simulink model "FSAC2021"  (R2014a)
settings: Solver=FixedStepDiscrete  StartTime=0.0  StopTime=inf  FixedStep=0.0005  RelTol=1e-3
model workspace (MAT data in the model file):
  MCOS : class17 (value not decoded)
  MCOS : class17 (value not decoded)
  MCOS : class17 (value not decoded)
  MCOS : class17 (value not decoded)
  MCOS : class17 (value not decoded)
  MCOS : class17 (value not decoded)
  MCOS : class17 (value not decoded)
  MCOS : class17 (value not decoded)
  MCOS : class17 (value not decoded)
  MCOS : class17 (value not decoded)
  MCOS : class17 (value not decoded)
  MCOS : class17 (value not decoded)
  MCOS : class17 (value not decoded)
  MCOS : class17 (value not decoded)
  MCOS : class17 (value not decoded)
  MCOS : class17 (value not decoded)
  MCOS : class17 (value not decoded)
  MCOS : class17 (value not decoded)
  MCOS : class17 (value not decoded)
  BUZZER_START = 1
  MCOS : class17 (value not decoded)
  MCOS : class17 (value not decoded)
  MCOS : class17 (value not decoded)
  MCOS : class17 (value not decoded)
  MCOS : class17 (value not decoded)
  MCOS : class17 (value not decoded)
  MCOS : class17 (value not decoded)
  MCOS : class17 (value not decoded)
  MCOS : class17 (value not decoded)
  MCOS : class17 (value not decoded)
  MCOS : class17 (value not decoded)
  MCOS : class17 (value not decoded)
  MCOS : class17 (value not decoded)
  MCOS : class17 (value not decoded)
  MCOS : class17 (value not decoded)
  MCOS : class17 (value not decoded)
  MCOS : class17 (value not decoded)
  MCOS : class17 (value not decoded)
  MCOS : class17 (value not decoded)
  MCOS : class17 (value not decoded)
  MCOS : class17 (value not decoded)
  MCOS : class17 (value not decoded)
  MCOS : class17 (value not decoded)
  MCOS : class17 (value not decoded)
  MCOS : class17 (value not decoded)
  MCOS : class17 (value not decoded)
  MCOS : class17 (value not decoded)
  MCOS : class17 (value not decoded)
  MCOS : class17 (value not decoded)
  MCOS : class17 (value not decoded)
  MCOS : class17 (value not decoded)
  MCOS : class17 (value not decoded)
  MCOS : class17 (value not decoded)
  MCOS : class17 (value not decoded)
  MCOS : class17 (value not decoded)
  MCOS : class17 (value not decoded)
  MCOS : class17 (value not decoded)
  MCOS : class17 (value not decoded)
  Brake = 11
  MCOS : class17 (value not decoded)
  MCOS : class17 (value not decoded)
  MCOS : class17 (value not decoded)
  MCOS : class17 (value not decoded)
  MCOS : class17 (value not decoded)
  MCOS : class17 (value not decoded)
  MCOS : class17 (value not decoded)
  MCOS : class17 (value not decoded)
  Sensor_Acc_b = 101.85
  Sensor_Acc_k = -0.0185
  Str_Sen_Orig_Angle = -341
  MCOS : class17 (value not decoded)
  Tire_D = 0.47
  T = 0.05
libraries: simulink x396, ec55xxlib x126
(part 8 of 17)

== system FSAC2021/CAN_SEND/Subsystem1/MOTEC_ENCODER1/Str_Encoder1 ==
  Str_Encoder1 : Inport
  Str_Encoder1Ron : Rounding  Operator=round
  Str_Encoder1_1sat : Saturate  UpperLimit=255  LowerLimit=0
  Str_Encoder1_Convert : DataTypeConversion  OutDataTypeStr=uint8
  Str_Encoder1_Convert1 : DataTypeConversion  OutDataTypeStr=uint32
  Str_Encoder1_D : Product  Inputs=*/
  Str_Encoder1_F : Constant  OutDataTypeStr=single
  Str_Encoder1_L : simulink/Logic and Bit Operations/Bitwise Operator  logicop=AND  UseBitMask=on  BitMask=255  BitMaskRealWorld=Stored Integer
  Str_Encoder1_O : Constant  Value=0  OutDataTypeStr=single
  Str_Encoder1_S : ArithShift
  Str_Encoder1_sat : Saturate  UpperLimit=255  LowerLimit=0
  Str_Encoder1_st : Sum  Inputs=+-
  output1 : Outport
  wires:
  Str_Encoder1/1 -> Str_Encoder1_sat/1
  Str_Encoder1_sat/1 -> Str_Encoder1_st/1
  Str_Encoder1_O/1 -> Str_Encoder1_st/2
  Str_Encoder1_st/1 -> Str_Encoder1_D/1
  Str_Encoder1_F/1 -> Str_Encoder1_D/2
  Str_Encoder1_D/1 -> Str_Encoder1Ron/1
  Str_Encoder1Ron/1 -> Str_Encoder1_S/1
  Str_Encoder1_S/1 -> Str_Encoder1_1sat/1
  Str_Encoder1_1sat/1 -> Str_Encoder1_Convert1/1
  Str_Encoder1_Convert1/1 -> Str_Encoder1_L/1
  Str_Encoder1_L/1 -> Str_Encoder1_Convert/1
  Str_Encoder1_Convert/1 -> output1/1

== system FSAC2021/CAN_SEND/Subsystem1/MOTEC_ENCODER1/Str_Encoder2 ==
  Str_Encoder2 : Inport
  Str_Encoder2Ron : Rounding  Operator=round
  Str_Encoder2_1sat : Saturate  UpperLimit=255  LowerLimit=0
  Str_Encoder2_Convert : DataTypeConversion  OutDataTypeStr=uint8
  Str_Encoder2_Convert1 : DataTypeConversion  OutDataTypeStr=uint32
  Str_Encoder2_D : Product  Inputs=*/
  Str_Encoder2_F : Constant  OutDataTypeStr=single
  Str_Encoder2_L : simulink/Logic and Bit Operations/Bitwise Operator  logicop=AND  UseBitMask=on  BitMask=255  BitMaskRealWorld=Stored Integer
  Str_Encoder2_O : Constant  Value=0  OutDataTypeStr=single
  Str_Encoder2_S : ArithShift
  Str_Encoder2_sat : Saturate  UpperLimit=255  LowerLimit=0
  Str_Encoder2_st : Sum  Inputs=+-
  output2 : Outport
  wires:
  Str_Encoder2/1 -> Str_Encoder2_sat/1
  Str_Encoder2_sat/1 -> Str_Encoder2_st/1
  Str_Encoder2_O/1 -> Str_Encoder2_st/2
  Str_Encoder2_st/1 -> Str_Encoder2_D/1
  Str_Encoder2_F/1 -> Str_Encoder2_D/2
  Str_Encoder2_D/1 -> Str_Encoder2Ron/1
  Str_Encoder2Ron/1 -> Str_Encoder2_S/1
  Str_Encoder2_S/1 -> Str_Encoder2_1sat/1
  Str_Encoder2_1sat/1 -> Str_Encoder2_Convert1/1
  Str_Encoder2_Convert1/1 -> Str_Encoder2_L/1
  Str_Encoder2_L/1 -> Str_Encoder2_Convert/1
  Str_Encoder2_Convert/1 -> output2/1

== system FSAC2021/CAN_SEND/Subsystem1/MOTEC_ENCODER1/Str_Encoder3 ==
  Str_Encoder3 : Inport
  Str_Encoder3Ron : Rounding  Operator=round
  Str_Encoder3_1sat : Saturate  UpperLimit=255  LowerLimit=0
  Str_Encoder3_Convert : DataTypeConversion  OutDataTypeStr=uint8
  Str_Encoder3_Convert1 : DataTypeConversion  OutDataTypeStr=uint32
  Str_Encoder3_D : Product  Inputs=*/
  Str_Encoder3_F : Constant  OutDataTypeStr=single
  Str_Encoder3_L : simulink/Logic and Bit Operations/Bitwise Operator  logicop=AND  UseBitMask=on  BitMask=255  BitMaskRealWorld=Stored Integer
  Str_Encoder3_O : Constant  Value=0  OutDataTypeStr=single
  Str_Encoder3_S : ArithShift
  Str_Encoder3_sat : Saturate  UpperLimit=255  LowerLimit=0
  Str_Encoder3_st : Sum  Inputs=+-
  output3 : Outport
  wires:
  Str_Encoder3/1 -> Str_Encoder3_sat/1
  Str_Encoder3_sat/1 -> Str_Encoder3_st/1
  Str_Encoder3_O/1 -> Str_Encoder3_st/2
  Str_Encoder3_st/1 -> Str_Encoder3_D/1
  Str_Encoder3_F/1 -> Str_Encoder3_D/2
  Str_Encoder3_D/1 -> Str_Encoder3Ron/1
  Str_Encoder3Ron/1 -> Str_Encoder3_S/1
  Str_Encoder3_S/1 -> Str_Encoder3_1sat/1
  Str_Encoder3_1sat/1 -> Str_Encoder3_Convert1/1
  Str_Encoder3_Convert1/1 -> Str_Encoder3_L/1
  Str_Encoder3_L/1 -> Str_Encoder3_Convert/1
  Str_Encoder3_Convert/1 -> output3/1

== system FSAC2021/CAN_SEND/Subsystem1/MOTEC_ENCODER1/Str_Encoder4 ==
  Str_Encoder4 : Inport
  Str_Encoder4Ron : Rounding  Operator=round
  Str_Encoder4_1sat : Saturate  UpperLimit=255  LowerLimit=0
  Str_Encoder4_Convert : DataTypeConversion  OutDataTypeStr=uint8
  Str_Encoder4_Convert1 : DataTypeConversion  OutDataTypeStr=uint32
  Str_Encoder4_D : Product  Inputs=*/
  Str_Encoder4_F : Constant  OutDataTypeStr=single
  Str_Encoder4_L : simulink/Logic and Bit Operations/Bitwise Operator  logicop=AND  UseBitMask=on  BitMask=255  BitMaskRealWorld=Stored Integer
  Str_Encoder4_O : Constant  Value=0  OutDataTypeStr=single
  Str_Encoder4_S : ArithShift
  Str_Encoder4_sat : Saturate  UpperLimit=255  LowerLimit=0
  Str_Encoder4_st : Sum  Inputs=+-
  output4 : Outport
  wires:
  Str_Encoder4/1 -> Str_Encoder4_sat/1
  Str_Encoder4_sat/1 -> Str_Encoder4_st/1
  Str_Encoder4_O/1 -> Str_Encoder4_st/2
  Str_Encoder4_st/1 -> Str_Encoder4_D/1
  Str_Encoder4_F/1 -> Str_Encoder4_D/2
  Str_Encoder4_D/1 -> Str_Encoder4Ron/1
  Str_Encoder4Ron/1 -> Str_Encoder4_S/1
  Str_Encoder4_S/1 -> Str_Encoder4_1sat/1
  Str_Encoder4_1sat/1 -> Str_Encoder4_Convert1/1
  Str_Encoder4_Convert1/1 -> Str_Encoder4_L/1
  Str_Encoder4_L/1 -> Str_Encoder4_Convert/1
  Str_Encoder4_Convert/1 -> output4/1

== system FSAC2021/CAN_SEND/Subsystem1/MOTEC_ENCODER1/Str_Encoder5 ==
  Str_Encoder5 : Inport
  Str_Encoder5Ron : Rounding  Operator=round
  Str_Encoder5_1sat : Saturate  UpperLimit=255  LowerLimit=0
  Str_Encoder5_Convert : DataTypeConversion  OutDataTypeStr=uint8
  Str_Encoder5_Convert1 : DataTypeConversion  OutDataTypeStr=uint32
  Str_Encoder5_D : Product  Inputs=*/
  Str_Encoder5_F : Constant  OutDataTypeStr=single
  Str_Encoder5_L : simulink/Logic and Bit Operations/Bitwise Operator  logicop=AND  UseBitMask=on  BitMask=255  BitMaskRealWorld=Stored Integer
  Str_Encoder5_O : Constant  Value=0  OutDataTypeStr=single
  Str_Encoder5_S : ArithShift
  Str_Encoder5_sat : Saturate  UpperLimit=255  LowerLimit=0
  Str_Encoder5_st : Sum  Inputs=+-
  output5 : Outport
  wires:
  Str_Encoder5/1 -> Str_Encoder5_sat/1
  Str_Encoder5_sat/1 -> Str_Encoder5_st/1
  Str_Encoder5_O/1 -> Str_Encoder5_st/2
  Str_Encoder5_st/1 -> Str_Encoder5_D/1
  Str_Encoder5_F/1 -> Str_Encoder5_D/2
  Str_Encoder5_D/1 -> Str_Encoder5Ron/1
  Str_Encoder5Ron/1 -> Str_Encoder5_S/1
  Str_Encoder5_S/1 -> Str_Encoder5_1sat/1
  Str_Encoder5_1sat/1 -> Str_Encoder5_Convert1/1
  Str_Encoder5_Convert1/1 -> Str_Encoder5_L/1
  Str_Encoder5_L/1 -> Str_Encoder5_Convert/1
  Str_Encoder5_Convert/1 -> output5/1

== system FSAC2021/CAN_SEND/Subsystem1/MOTEC_ENCODER1/Str_Encoder6 ==
  Str_Encoder6 : Inport
  Str_Encoder6Ron : Rounding  Operator=round
  Str_Encoder6_1sat : Saturate  UpperLimit=255  LowerLimit=0
  Str_Encoder6_Convert : DataTypeConversion  OutDataTypeStr=uint8
  Str_Encoder6_Convert1 : DataTypeConversion  OutDataTypeStr=uint32
  Str_Encoder6_D : Product  Inputs=*/
  Str_Encoder6_F : Constant  OutDataTypeStr=single
  Str_Encoder6_L : simulink/Logic and Bit Operations/Bitwise Operator  logicop=AND  UseBitMask=on  BitMask=255  BitMaskRealWorld=Stored Integer
  Str_Encoder6_O : Constant  Value=0  OutDataTypeStr=single
  Str_Encoder6_S : ArithShift
  Str_Encoder6_sat : Saturate  UpperLimit=255  LowerLimit=0
  Str_Encoder6_st : Sum  Inputs=+-
  output6 : Outport
  wires:
  Str_Encoder6/1 -> Str_Encoder6_sat/1
  Str_Encoder6_sat/1 -> Str_Encoder6_st/1
  Str_Encoder6_O/1 -> Str_Encoder6_st/2
  Str_Encoder6_st/1 -> Str_Encoder6_D/1
  Str_Encoder6_F/1 -> Str_Encoder6_D/2
  Str_Encoder6_D/1 -> Str_Encoder6Ron/1
  Str_Encoder6Ron/1 -> Str_Encoder6_S/1
  Str_Encoder6_S/1 -> Str_Encoder6_1sat/1
  Str_Encoder6_1sat/1 -> Str_Encoder6_Convert1/1
  Str_Encoder6_Convert1/1 -> Str_Encoder6_L/1
  Str_Encoder6_L/1 -> Str_Encoder6_Convert/1
  Str_Encoder6_Convert/1 -> output6/1

== system FSAC2021/CAN_SEND/Subsystem1/MOTEC_NMT/NMT_nodectrl ==
  NMT_nodectrl : Inport
  NMT_nodectrlRon : Rounding  Operator=round
  NMT_nodectrl_1sat : Saturate  UpperLimit=255  LowerLimit=0
  NMT_nodectrl_Convert : DataTypeConversion  OutDataTypeStr=uint8
  NMT_nodectrl_Convert1 : DataTypeConversion  OutDataTypeStr=uint32
  NMT_nodectrl_D : Product  Inputs=*/
  NMT_nodectrl_F : Constant  OutDataTypeStr=single
  NMT_nodectrl_L : simulink/Logic and Bit Operations/Bitwise Operator  logicop=AND  UseBitMask=on  BitMask=255  BitMaskRealWorld=Stored Integer
  NMT_nodectrl_O : Constant  Value=0  OutDataTypeStr=single
  NMT_nodectrl_S : ArithShift
  NMT_nodectrl_sat : Saturate  UpperLimit=255  LowerLimit=0
  NMT_nodectrl_st : Sum  Inputs=+-
  output2 : Outport
  wires:
  NMT_nodectrl/1 -> NMT_nodectrl_sat/1
  NMT_nodectrl_sat/1 -> NMT_nodectrl_st/1
  NMT_nodectrl_O/1 -> NMT_nodectrl_st/2
  NMT_nodectrl_st/1 -> NMT_nodectrl_D/1
  NMT_nodectrl_F/1 -> NMT_nodectrl_D/2
  NMT_nodectrl_D/1 -> NMT_nodectrlRon/1
  NMT_nodectrlRon/1 -> NMT_nodectrl_S/1
  NMT_nodectrl_S/1 -> NMT_nodectrl_1sat/1
  NMT_nodectrl_1sat/1 -> NMT_nodectrl_Convert1/1
  NMT_nodectrl_Convert1/1 -> NMT_nodectrl_L/1
  NMT_nodectrl_L/1 -> NMT_nodectrl_Convert/1
  NMT_nodectrl_Convert/1 -> output2/1

== system FSAC2021/CAN_SEND/Subsystem1/MOTEC_NMT/NMT_nodeorder ==
  NMT_nodeorder : Inport
  NMT_nodeorderRon : Rounding  Operator=round
  NMT_nodeorder_1sat : Saturate  UpperLimit=255  LowerLimit=0
  NMT_nodeorder_Convert : DataTypeConversion  OutDataTypeStr=uint8
  NMT_nodeorder_Convert1 : DataTypeConversion  OutDataTypeStr=uint32
  NMT_nodeorder_D : Product  Inputs=*/
  NMT_nodeorder_F : Constant  OutDataTypeStr=single
  NMT_nodeorder_L : simulink/Logic and Bit Operations/Bitwise Operator  logicop=AND  UseBitMask=on  BitMask=255  BitMaskRealWorld=Stored Integer
  NMT_nodeorder_O : Constant  Value=0  OutDataTypeStr=single
  NMT_nodeorder_S : ArithShift
  NMT_nodeorder_sat : Saturate  UpperLimit=255  LowerLimit=0
  NMT_nodeorder_st : Sum  Inputs=+-
  output1 : Outport
  wires:
  NMT_nodeorder/1 -> NMT_nodeorder_sat/1
  NMT_nodeorder_sat/1 -> NMT_nodeorder_st/1
  NMT_nodeorder_O/1 -> NMT_nodeorder_st/2
  NMT_nodeorder_st/1 -> NMT_nodeorder_D/1
  NMT_nodeorder_F/1 -> NMT_nodeorder_D/2
  NMT_nodeorder_D/1 -> NMT_nodeorderRon/1
  NMT_nodeorderRon/1 -> NMT_nodeorder_S/1
  NMT_nodeorder_S/1 -> NMT_nodeorder_1sat/1
  NMT_nodeorder_1sat/1 -> NMT_nodeorder_Convert1/1
  NMT_nodeorder_Convert1/1 -> NMT_nodeorder_L/1
  NMT_nodeorder_L/1 -> NMT_nodeorder_Convert/1
  NMT_nodeorder_Convert/1 -> output1/1

== system FSAC2021/Controller/200ms_Duty/Light_Subsystem/BLINK  ==
  Action Port : ActionPort  ActionType=else
  Data Type Conversion : DataTypeConversion  OutDataTypeStr=uint8
  Logical Operator : Logic  Operator=NOT  AllPortsSameDT=off  OutDataTypeStr=boolean
  Unit Delay : UnitDelay  SampleTime=-1
  Out1 : Outport
  wires:
  Logical Operator/1 -> Data Type Conversion/1
  Data Type Conversion/1 -> Unit Delay/1, Out1/1
  Unit Delay/1 -> Logical Operator/1

== system FSAC2021/Controller/200ms_Duty/Light_Subsystem/OFF ==
  Action Port : ActionPort  ActionType=elseif
  Constant : Constant  OutDataTypeStr=uint8
  Out1 : Outport
  wires:
  Constant/1 -> Out1/1

== system FSAC2021/Controller/200ms_Duty/Light_Subsystem/ON ==
  Action Port : ActionPort  ActionType=then
  Constant : Constant  Value=0  OutDataTypeStr=uint8
  Out1 : Outport
  wires:
  Constant/1 -> Out1/1

== system FSAC2021/Controller/200ms_Duty/Light_Subsystem1/BLINK ==
  Action Port : ActionPort  ActionType=else
  Data Type Conversion : DataTypeConversion  OutDataTypeStr=uint8
  Logical Operator : Logic  Operator=NOT  AllPortsSameDT=off  OutDataTypeStr=boolean
  Unit Delay : UnitDelay  SampleTime=-1
  Out1 : Outport
  wires:
  Unit Delay/1 -> Logical Operator/1
  Data Type Conversion/1 -> Out1/1, Unit Delay/1
  Logical Operator/1 -> Data Type Conversion/1

== system FSAC2021/Controller/200ms_Duty/Light_Subsystem1/OFF ==
  Action Port : ActionPort  ActionType=elseif
  Constant : Constant  OutDataTypeStr=uint8
  Out1 : Outport
  wires:
  Constant/1 -> Out1/1

== system FSAC2021/Controller/200ms_Duty/Light_Subsystem1/ON ==
  Action Port : ActionPort  ActionType=then
  Constant : Constant  Value=0  OutDataTypeStr=uint8
  Out1 : Outport
  wires:
  Constant/1 -> Out1/1

== system FSAC2021/Controller/200ms_Duty/Light_Subsystem2/EBS_Horn ==
  Action Port : ActionPort  ActionType=else
  Chart : Stateflow chart  TreatAsAtomicUnit=on
  Buzzer_Pin : Outport
  Buzzer_Overflag : Outport  Port=2
  wires:
  Chart/1(Buzzer_Pin) -> Buzzer_Pin/1
  Chart/2(Buzzer_Overflag) -> Buzzer_Overflag/1

== system FSAC2021/Controller/200ms_Duty/Light_Subsystem2/Start_Horn ==
  Action Port : ActionPort  ActionType=elseif
  Chart : Stateflow chart  TreatAsAtomicUnit=on
  Out1 : Outport
  wires:
  Chart/1(Buzzer_Pin) -> Out1/1

== system FSAC2021/Controller/200ms_Duty/Light_Subsystem2/off ==
  Action Port : ActionPort  ActionType=then
  Constant : Constant  Value=0  OutDataTypeStr=uint8
  Out1 : Outport
  wires:
  Constant/1 -> Out1/1

== system FSAC2021/Controller/50ms_Duty/Subsystem/Subsystem ==
  acc : Inport
  Enable : EnablePort
  Gain : Gain  Gain=15
  Saturation : Saturate  UpperLimit=1500  LowerLimit=0
  Acc_Cmd : Outport
  wires:
  acc/1 -> Gain/1
  Gain/1 -> Saturation/1
  Saturation/1 -> Acc_Cmd/1

== system FSAC2021/Controller/50ms_Duty/Subsystem/Subsystem1 ==
  IPC_Acc_Cmd : Inport
  EBS_Failure : Inport  Port=2
  IPC_Brk_Cmd : Inport  Port=3
  IPC_Str_Cmd : Inport  Port=4
  Enable : EnablePort
  Gain : Gain  Gain=15
  Redundant_Brk_Cmd : Constant  Value=100  OutDataTypeStr=single
  Switch2 : Switch  Criteria=u2 ~= 0  Threshold=5
  Terminator : Terminator
  Brk_Cmd : Outport
  Str_Cmd : Outport  Port=2
  Acc_Cmd : Outport  Port=3
  wires:
  IPC_Str_Cmd/1 -> Str_Cmd/1
  Redundant_Brk_Cmd/1 -> Switch2/1
  EBS_Failure/1 -> Switch2/2
  IPC_Acc_Cmd/1 -> Gain/1
  Gain/1 -> Acc_Cmd/1
  IPC_Brk_Cmd/1 -> Brk_Cmd/1
  Switch2/1 -> Terminator/1

== system FSAC2021/Controller/50ms_Duty/Subsystem/Subsystem2 ==
  Enable : EnablePort
  Chart : Stateflow chart  TreatAsAtomicUnit=on
  ACC : Outport
  SteerCmd : Outport  Port=2
  Mission_Flag : Outport  Port=3
  wires:
  Chart/1(Mission_Flag) -> Mission_Flag/1
  Chart/3(ACC) -> ACC/1
  Chart/2(SteerCmd) -> SteerCmd/1

== system FSAC2021/Controller/BCU_Controller/Brk_Move/Enabled Subsystem ==
  Enable : EnablePort
  Angle2Pulses : Subsystem  TreatAsAtomicUnit=on
  Constant : Constant  Value=BRK_Engaged_Angle  OutDataTypeStr=int8
  Engaged_Pulses : Outport
  Engaged_Angle : Outport  Port=2
  wires:
  Angle2Pulses/1(Pulses) -> Engaged_Pulses/1
  Constant/1 -> Angle2Pulses/1(Angle), Engaged_Angle/1

== system FSAC2021/Controller/BCU_Controller/Brk_Move/Enabled Subsystem1 ==
  Engaged_Angle : Inport
  Enable : EnablePort
  Angle2Pulses : Subsystem  TreatAsAtomicUnit=on
  Gain : Gain  Gain=-1  ParamDataTypeStr=int8  OutDataTypeStr=int8
  ToZero_Pulses : Outport
  wires:
  Gain/1 -> Angle2Pulses/1(Angle)
  Angle2Pulses/1(Pulses) -> ToZero_Pulses/1
  Engaged_Angle/1 -> Gain/1

== system FSAC2021/Controller/BCU_Controller/Brk_Move/Enabled Subsystem2 ==
  note: 制动百分比
  note: 电机反转
  Brk_Prop : Inport
  Enable : EnablePort
  Angle2Pulses : Subsystem  TreatAsAtomicUnit=on
  Brk_Prop2Angle : Gain  Gain=Brk_Prop2Angle
  Gain : Gain  Gain=-1  ParamDataTypeStr=int8  OutDataTypeStr=single
  Move_Pulses : Outport
  wires:
  Gain/1 -> Angle2Pulses/1(Angle)
  Brk_Prop/1 -> Brk_Prop2Angle/1
  Brk_Prop2Angle/1 -> Gain/1
  Angle2Pulses/1(Pulses) -> Move_Pulses/1

== system FSAC2021/DIAG/DIAG/CAN_NODE_LOSTCOM/B_M_S_Check ==
  Brake_Node : Inport
  Motec_Node : Inport  Port=2
  RES_Node : Inport  Port=3
  Enable : EnablePort
  Chart : Stateflow chart  TreatAsAtomicUnit=on
      settings: RTWSystemCode=Reusable function
  Chart1 : Stateflow chart  TreatAsAtomicUnit=on
      settings: RTWSystemCode=Reusable function
  Logical Operator : Logic  AllPortsSameDT=off  OutDataTypeStr=boolean
  MeaModule1 : ec55xxlib/RapidECU_U2/11Calibration/MeaModule  signal=BRAKE
  MeaModule2 : ec55xxlib/RapidECU_U2/11Calibration/MeaModule  signal=MOTEC
  Node_Lost_Flag : Outport
  wires:
  Logical Operator/1 -> Node_Lost_Flag/1
  Brake_Node/1 -> Chart1/1(Input)
  MeaModule1/1 -> Logical Operator/1
  MeaModule2/1 -> Logical Operator/2
  Motec_Node/1 -> Chart/1(Input)
  Chart/1(Output) -> MeaModule2/1
  Chart1/1(Output) -> MeaModule1/1

== system FSAC2021/DIAG/DIAG/CAN_NODE_LOSTCOM/Subsystem ==
  Motor_Node : Inport
  Enable : EnablePort
  Chart4 : Stateflow chart  TreatAsAtomicUnit=on
      settings: RTWSystemCode=Reusable function
  MeaModule1 : ec55xxlib/RapidECU_U2/11Calibration/MeaModule  signal=motor
  Node_Lost_Flag : Outport
  wires:
  MeaModule1/1 -> Node_Lost_Flag/1
  Motor_Node/1 -> Chart4/1(Input)
  Chart4/1(Output) -> MeaModule1/1

== system FSAC2021/DIAG/DIAG/CAN_NODE_LOSTCOM/Subsystem1 ==
  StrSr_Node : Inport
  BMS_Node : Inport  Port=2
  AMI_Node : Inport  Port=3
  Chart2 : Stateflow chart  TreatAsAtomicUnit=on
      settings: RTWSystemCode=Reusable function
  Chart3 : Stateflow chart  TreatAsAtomicUnit=on
      settings: RTWSystemCode=Reusable function
  Chart4 : Stateflow chart  TreatAsAtomicUnit=on
      settings: RTWSystemCode=Reusable function
  Logical Operator : Logic  Inputs=3  AllPortsSameDT=off  OutDataTypeStr=boolean
  MeaModule3 : ec55xxlib/RapidECU_U2/11Calibration/MeaModule  signal=STRSNR
  MeaModule4 : ec55xxlib/RapidECU_U2/11Calibration/MeaModule  signal=BMS
  MeaModule5 : ec55xxlib/RapidECU_U2/11Calibration/MeaModule  signal=AMI_NODE
  Out1 : Outport
  wires:
  StrSr_Node/1 -> Chart2/1(Input)
  Chart2/1(Output) -> MeaModule3/1
  Chart4/1(Output) -> MeaModule5/1
  Chart3/1(Output) -> MeaModule4/1
  BMS_Node/1 -> Chart3/1(Input)
  AMI_Node/1 -> Chart4/1(Input)
  MeaModule3/1 -> Logical Operator/1
  MeaModule4/1 -> Logical Operator/2
  MeaModule5/1 -> Logical Operator/3
  Logical Operator/1 -> Out1/1

== system FSAC2021/DIAG/DIAG/TS_Diag/Subsystem ==
  Compare_Volt_mv : Inport
  Enable : EnablePort
  Compare To Constant3 : simulink/Logic and Bit Operations/Compare To Constant  relop=<  const=2  OutDataTypeStr=boolean
  TS_Error : Outport
  wires:
  Compare_Volt_mv/1 -> Compare To Constant3/1
  Compare To Constant3/1 -> TS_Error/1

== system FSAC2021/DIAG/DIAG/TS_Diag/Subsystem1 ==
  Compare_Volt_mv : Inport
  Enable : EnablePort
  Compare To Constant3 : simulink/Logic and Bit Operations/Compare To Constant  relop=<  const=2  OutDataTypeStr=boolean
  TS_Error : Outport
  wires:
  Compare_Volt_mv/1 -> Compare To Constant3/1
  Compare To Constant3/1 -> TS_Error/1

== system FSAC2021/DIAG/DIAG/TS_Diag/Subsystem2 ==
  Compare_Volt_mv : Inport
  Enable : EnablePort
  Compare To Constant3 : simulink/Logic and Bit Operations/Compare To Constant  relop=<  const=2  OutDataTypeStr=boolean
  TS_Error : Outport
  wires:
  Compare_Volt_mv/1 -> Compare To Constant3/1
  Compare To Constant3/1 -> TS_Error/1

== system FSAC2021/Input_Process/KL_Sig_Process/Whl_Spd_Process/LPF ==
  note: y(t) = K*u(t) + (1-K)*y(t-1) = y(t-1) + K*[u(t)-y(t-1)]
      | 其中，K=dT/T，K一般介于0~1之间，dT是运行步长，T是时间常数；u是输入信号；y是输出信号。
  Filter : Inport
  Add : Sum  Inputs=+-  AccumDataTypeStr=single
  Add1 : Sum  AccumDataTypeStr=single
  Constant : Constant  Value=Filter_Factor
  Product : Product  OutDataTypeStr=single
  Unit Delay : UnitDelay  InitialCondition=1  SampleTime=-1
  Filtered : Outport
  wires:
  Add1/1 -> Unit Delay/1, Filtered/1
  Filter/1 -> Add/1
  Unit Delay/1 -> Add1/2, Add/2
  Add/1 -> Product/2
  Constant/1 -> Product/1
  Product/1 -> Add1/1

== system FSAC2021/Input_Process/KL_Sig_Process/Whl_Spd_Process/LPF1 ==
  note: y(t) = K*u(t) + (1-K)*y(t-1) = y(t-1) + K*[u(t)-y(t-1)]
      | 其中，K=dT/T，K一般介于0~1之间，dT是运行步长，T是时间常数；u是输入信号；y是输出信号。
  Filter : Inport
  Add : Sum  Inputs=+-  AccumDataTypeStr=single
  Add1 : Sum  AccumDataTypeStr=single
  Constant : Constant  Value=Filter_Factor
  Product : Product  OutDataTypeStr=single
  Unit Delay : UnitDelay  InitialCondition=1  SampleTime=-1
  Filtered : Outport
  wires:
  Product/1 -> Add1/1
  Constant/1 -> Product/1
  Add/1 -> Product/2
  Unit Delay/1 -> Add/2, Add1/2
  Filter/1 -> Add/1
  Add1/1 -> Filtered/1, Unit Delay/1

== system FSAC2021/Input_Process/KL_Sig_Process/Whl_Spd_Process/LPF2 ==
  note: y(t) = K*u(t) + (1-K)*y(t-1) = y(t-1) + K*[u(t)-y(t-1)]
      | 其中，K=dT/T，K一般介于0~1之间，dT是运行步长，T是时间常数；u是输入信号；y是输出信号。
  Filter : Inport
  Add : Sum  Inputs=+-  AccumDataTypeStr=single
  Add1 : Sum  AccumDataTypeStr=single
  Constant : Constant  Value=Filter_Factor
  Product : Product  OutDataTypeStr=single
  Unit Delay : UnitDelay  InitialCondition=1  SampleTime=-1
  Filtered : Outport
  wires:
  Add1/1 -> Unit Delay/1, Filtered/1
  Filter/1 -> Add/1
  Unit Delay/1 -> Add1/2, Add/2
  Add/1 -> Product/2
  Constant/1 -> Product/1
  Product/1 -> Add1/1

== system FSAC2021/Input_Process/KL_Sig_Process/Whl_Spd_Process/LPF3 ==
  note: y(t) = K*u(t) + (1-K)*y(t-1) = y(t-1) + K*[u(t)-y(t-1)]
      | 其中，K=dT/T，K一般介于0~1之间，dT是运行步长，T是时间常数；u是输入信号；y是输出信号。
  Filter : Inport
  Add : Sum  Inputs=+-  AccumDataTypeStr=single
  Add1 : Sum  AccumDataTypeStr=single
  Constant : Constant  Value=Filter_Factor
  Product : Product  OutDataTypeStr=single
  Unit Delay : UnitDelay  InitialCondition=1  SampleTime=-1
  Filtered : Outport
  wires:
  Product/1 -> Add1/1
  Constant/1 -> Product/1
  Add/1 -> Product/2
  Unit Delay/1 -> Add/2, Add1/2
  Filter/1 -> Add/1
  Add1/1 -> Filtered/1, Unit Delay/1

== system FSAC2021/Input_Process/KL_Sig_Process/Whl_Spd_Process/Whl2Veh_Spd_Trans ==
  Wheel_speed_rightrear_wheel : Inport
  Wheel_speed_right_front_wheel : Inport  Port=2
  Wheel_speed_leftrear_wheel : Inport  Port=3
  Wheel_speed_leftfront_wheel : Inport  Port=4
  Round : Subsystem  TreatAsAtomicUnit=on
  Wheel_Mean : Subsystem
  rpm2km_h : Subsystem
  Vel_Speed : Outport
  wires:
  Wheel_speed_leftfront_wheel/1 -> Wheel_Mean/4(Wheel_speed_leftfront_wheel)
  Wheel_speed_leftrear_wheel/1 -> Wheel_Mean/3(Wheel_speed_leftrear_wheel)
  Wheel_speed_rightrear_wheel/1 -> Wheel_Mean/1(Wheel_speed_rightrear_wheel)
  Wheel_speed_right_front_wheel/1 -> Wheel_Mean/2(Wheel_speed_right_front_wheel)
  Wheel_Mean/1(Out1) -> rpm2km_h/1(rpm)
  rpm2km_h/1(kmph) -> Round/1(Origin_Precision)
  Round/1(Two_Precision) -> Vel_Speed/1

== system FSAC2021/Input_Process/KL_Sig_Process/Whl_Spd_Process/Whl_Spd_Hz2RPM ==
  Whl_Spd_Hz : Inport  OutDataTypeStr=uint32
  Constant : Constant  Value=FTeeth_Wheel  OutDataTypeStr=single
  Divide : Product  Inputs=*/
  rps2rpm : Gain  Gain=60  ParamDataTypeStr=uint16  OutDataTypeStr=single
  Whl_Spd_RPM : Outport
  wires:
  Divide/1 -> rps2rpm/1
  Constant/1 -> Divide/2
  Whl_Spd_Hz/1 -> Divide/1
  rps2rpm/1 -> Whl_Spd_RPM/1

== system FSAC2021/Input_Process/KL_Sig_Process/Whl_Spd_Process/Whl_Spd_Hz2RPM1 ==
  Whl_Spd_Hz : Inport  OutDataTypeStr=uint32
  Constant : Constant  Value=FTeeth_Wheel  OutDataTypeStr=single
  Divide : Product  Inputs=*/
  rps2rpm : Gain  Gain=60  ParamDataTypeStr=uint16  OutDataTypeStr=single
  Whl_Spd_RPM : Outport
  wires:
  rps2rpm/1 -> Whl_Spd_RPM/1
  Whl_Spd_Hz/1 -> Divide/1
  Constant/1 -> Divide/2
  Divide/1 -> rps2rpm/1

== system FSAC2021/Input_Process/KL_Sig_Process/Whl_Spd_Process/Whl_Spd_Hz2RPM2 ==
  Whl_Spd_Hz : Inport  OutDataTypeStr=uint32
  Constant : Constant  Value=RTeeth_Wheel  OutDataTypeStr=single
  Divide : Product  Inputs=*/
  rps2rpm : Gain  Gain=60  ParamDataTypeStr=uint16  OutDataTypeStr=single
  Whl_Spd_RPM : Outport
  wires:
  Divide/1 -> rps2rpm/1
  Constant/1 -> Divide/2
  Whl_Spd_Hz/1 -> Divide/1
  rps2rpm/1 -> Whl_Spd_RPM/1

== system FSAC2021/Input_Process/KL_Sig_Process/Whl_Spd_Process/Whl_Spd_Hz2RPM3 ==
  Whl_Spd_Hz : Inport  OutDataTypeStr=uint32
  Constant : Constant  Value=RTeeth_Wheel  OutDataTypeStr=single
  Divide : Product  Inputs=*/
  rps2rpm : Gain  Gain=60  ParamDataTypeStr=uint16  OutDataTypeStr=single
  Whl_Spd_RPM : Outport
  wires:
  rps2rpm/1 -> Whl_Spd_RPM/1
  Whl_Spd_Hz/1 -> Divide/1
  Constant/1 -> Divide/2
  Divide/1 -> rps2rpm/1

== system FSAC2021/ROUTING/TO_ACAN/DV_driving_dynamics_1/Brake_hydr_actual ==
  Brake_hydr_actual : Inport
  Brake_hydr_actualRon : Rounding  Operator=round
  Brake_hydr_actual_1sat : Saturate  UpperLimit=255  LowerLimit=0
  Brake_hydr_actual_Convert : DataTypeConversion  OutDataTypeStr=uint8
  Brake_hydr_actual_Convert1 : DataTypeConversion  OutDataTypeStr=uint32
  Brake_hydr_actual_D : Product  Inputs=*/
  Brake_hydr_actual_F : Constant  OutDataTypeStr=single
  Brake_hydr_actual_L : simulink/Logic and Bit Operations/Bitwise Operator  logicop=AND  UseBitMask=on  BitMask=255  BitMaskRealWorld=Stored Integer
  Brake_hydr_actual_O : Constant  Value=0  OutDataTypeStr=single
  Brake_hydr_actual_S : ArithShift
  Brake_hydr_actual_sat : Saturate  UpperLimit=100  LowerLimit=0
  Brake_hydr_actual_st : Sum  Inputs=+-
  output5 : Outport
  wires:
  Brake_hydr_actual/1 -> Brake_hydr_actual_sat/1
  Brake_hydr_actual_sat/1 -> Brake_hydr_actual_st/1
  Brake_hydr_actual_O/1 -> Brake_hydr_actual_st/2
  Brake_hydr_actual_st/1 -> Brake_hydr_actual_D/1
  Brake_hydr_actual_F/1 -> Brake_hydr_actual_D/2
  Brake_hydr_actual_D/1 -> Brake_hydr_actualRon/1
  Brake_hydr_actualRon/1 -> Brake_hydr_actual_S/1
  Brake_hydr_actual_S/1 -> Brake_hydr_actual_1sat/1
  Brake_hydr_actual_1sat/1 -> Brake_hydr_actual_Convert1/1
  Brake_hydr_actual_Convert1/1 -> Brake_hydr_actual_L/1
  Brake_hydr_actual_L/1 -> Brake_hydr_actual_Convert/1
  Brake_hydr_actual_Convert/1 -> output5/1

== system FSAC2021/ROUTING/TO_ACAN/DV_driving_dynamics_1/Brake_hydr_target ==
  Brake_hydr_target : Inport
  Brake_hydr_targetRon : Rounding  Operator=round
  Brake_hydr_target_1sat : Saturate  UpperLimit=255  LowerLimit=0
  Brake_hydr_target_Convert : DataTypeConversion  OutDataTypeStr=uint8
  Brake_hydr_target_Convert1 : DataTypeConversion  OutDataTypeStr=uint32
  Brake_hydr_target_D : Product  Inputs=*/
  Brake_hydr_target_F : Constant  OutDataTypeStr=single
  Brake_hydr_target_L : simulink/Logic and Bit Operations/Bitwise Operator  logicop=AND  UseBitMask=on  BitMask=255  BitMaskRealWorld=Stored Integer
  Brake_hydr_target_O : Constant  Value=0  OutDataTypeStr=single
  Brake_hydr_target_S : ArithShift
  Brake_hydr_target_sat : Saturate  UpperLimit=100  LowerLimit=0
  Brake_hydr_target_st : Sum  Inputs=+-
  output6 : Outport
  wires:
  Brake_hydr_target/1 -> Brake_hydr_target_sat/1
  Brake_hydr_target_sat/1 -> Brake_hydr_target_st/1
  Brake_hydr_target_O/1 -> Brake_hydr_target_st/2
  Brake_hydr_target_st/1 -> Brake_hydr_target_D/1
  Brake_hydr_target_F/1 -> Brake_hydr_target_D/2
  Brake_hydr_target_D/1 -> Brake_hydr_targetRon/1
  Brake_hydr_targetRon/1 -> Brake_hydr_target_S/1
  Brake_hydr_target_S/1 -> Brake_hydr_target_1sat/1
  Brake_hydr_target_1sat/1 -> Brake_hydr_target_Convert1/1
  Brake_hydr_target_Convert1/1 -> Brake_hydr_target_L/1
  Brake_hydr_target_L/1 -> Brake_hydr_target_Convert/1
  Brake_hydr_target_Convert/1 -> output6/1

== system FSAC2021/ROUTING/TO_ACAN/DV_driving_dynamics_1/Motor_moment_actual ==
  Motor_moment_actual : Inport
  Motor_moment_actualABS : Abs
  Motor_moment_actualCS : ArithShift  BitShiftNumber=-8
  Motor_moment_actualConS : Constant  OutDataTypeStr=single
  Motor_moment_actualCosR : Constant  Value=0  OutDataTypeStr=uint8
  Motor_moment_actualROP : RelationalOperator  Operator=<  OutDataTypeStr=boolean
  Motor_moment_actualRon : Rounding  Operator=round
  Motor_moment_actualSW : Switch  Criteria=u2 ~= 0
  Motor_moment_actual_1sat : Saturate  UpperLimit=255  LowerLimit=0
  Motor_moment_actual_Convert : DataTypeConversion  OutDataTypeStr=uint8
  Motor_moment_actual_Convert1 : DataTypeConversion  OutDataTypeStr=uint32
  Motor_moment_actual_D : Product  Inputs=*/
  Motor_moment_actual_F : Constant  OutDataTypeStr=single
  Motor_moment_actual_L : simulink/Logic and Bit Operations/Bitwise Operator  logicop=AND  UseBitMask=on  BitMask=255  BitMaskRealWorld=Stored Integer
  Motor_moment_actual_O : Constant  Value=0  OutDataTypeStr=single
  Motor_moment_actual_S : ArithShift
  Motor_moment_actual_sat : Saturate  UpperLimit=100  LowerLimit=0
  Motor_moment_actual_st : Sum  Inputs=+-
  Motor_moment_actualsubcon : Sum  Inputs=+-
  output7 : Outport
  wires:
  Motor_moment_actual/1 -> Motor_moment_actual_sat/1
  Motor_moment_actual_sat/1 -> Motor_moment_actual_st/1
  Motor_moment_actual_O/1 -> Motor_moment_actual_st/2
  Motor_moment_actual_st/1 -> Motor_moment_actual_D/1
  Motor_moment_actual_F/1 -> Motor_moment_actual_D/2
  Motor_moment_actual_D/1 -> Motor_moment_actualRon/1
  Motor_moment_actualRon/1 -> Motor_moment_actualROP/1, Motor_moment_actualABS/1, Motor_moment_actualSW/3
  Motor_moment_actualCosR/1 -> Motor_moment_actualROP/2
  Motor_moment_actualConS/1 -> Motor_moment_actualCS/1
  Motor_moment_actualCS/1 -> Motor_moment_actualsubcon/1
  Motor_moment_actualABS/1 -> Motor_moment_actualsubcon/2
  Motor_moment_actualsubcon/1 -> Motor_moment_actualSW/1
  Motor_moment_actualROP/1 -> Motor_moment_actualSW/2
  Motor_moment_actualSW/1 -> Motor_moment_actual_S/1
  Motor_moment_actual_S/1 -> Motor_moment_actual_1sat/1
  Motor_moment_actual_1sat/1 -> Motor_moment_actual_Convert1/1
  Motor_moment_actual_Convert1/1 -> Motor_moment_actual_L/1
  Motor_moment_actual_L/1 -> Motor_moment_actual_Convert/1
  Motor_moment_actual_Convert/1 -> output7/1

== system FSAC2021/ROUTING/TO_ACAN/DV_driving_dynamics_1/Motor_moment_target ==
  Motor_moment_target : Inport
  Motor_moment_targetABS : Abs
  Motor_moment_targetCS : ArithShift  BitShiftNumber=-8
  Motor_moment_targetConS : Constant  OutDataTypeStr=single
  Motor_moment_targetCosR : Constant  Value=0  OutDataTypeStr=uint8
  Motor_moment_targetROP : RelationalOperator  Operator=<  OutDataTypeStr=boolean
  Motor_moment_targetRon : Rounding  Operator=round
  Motor_moment_targetSW : Switch  Criteria=u2 ~= 0
  Motor_moment_target_1sat : Saturate  UpperLimit=255  LowerLimit=0
  Motor_moment_target_Convert : DataTypeConversion  OutDataTypeStr=uint8
  Motor_moment_target_Convert1 : DataTypeConversion  OutDataTypeStr=uint32
  Motor_moment_target_D : Product  Inputs=*/
  Motor_moment_target_F : Constant  OutDataTypeStr=single
  Motor_moment_target_L : simulink/Logic and Bit Operations/Bitwise Operator  logicop=AND  UseBitMask=on  BitMask=255  BitMaskRealWorld=Stored Integer
  Motor_moment_target_O : Constant  Value=0  OutDataTypeStr=single
  Motor_moment_target_S : ArithShift
  Motor_moment_target_sat : Saturate  UpperLimit=100  LowerLimit=0
  Motor_moment_target_st : Sum  Inputs=+-
  Motor_moment_targetsubcon : Sum  Inputs=+-
  output8 : Outport
  wires:
  Motor_moment_target/1 -> Motor_moment_target_sat/1
  Motor_moment_target_sat/1 -> Motor_moment_target_st/1
  Motor_moment_target_O/1 -> Motor_moment_target_st/2
  Motor_moment_target_st/1 -> Motor_moment_target_D/1
  Motor_moment_target_F/1 -> Motor_moment_target_D/2
  Motor_moment_target_D/1 -> Motor_moment_targetRon/1
  Motor_moment_targetRon/1 -> Motor_moment_targetROP/1, Motor_moment_targetABS/1, Motor_moment_targetSW/3
  Motor_moment_targetCosR/1 -> Motor_moment_targetROP/2
  Motor_moment_targetConS/1 -> Motor_moment_targetCS/1
  Motor_moment_targetCS/1 -> Motor_moment_targetsubcon/1
  Motor_moment_targetABS/1 -> Motor_moment_targetsubcon/2
  Motor_moment_targetsubcon/1 -> Motor_moment_targetSW/1
  Motor_moment_targetROP/1 -> Motor_moment_targetSW/2
  Motor_moment_targetSW/1 -> Motor_moment_target_S/1
  Motor_moment_target_S/1 -> Motor_moment_target_1sat/1
  Motor_moment_target_1sat/1 -> Motor_moment_target_Convert1/1
  Motor_moment_target_Convert1/1 -> Motor_moment_target_L/1
  Motor_moment_target_L/1 -> Motor_moment_target_Convert/1
  Motor_moment_target_Convert/1 -> output8/1

== system FSAC2021/ROUTING/TO_ACAN/DV_driving_dynamics_1/Speeed_actual ==
  Speeed_actual : Inport
  Speeed_actualRon : Rounding  Operator=round
  Speeed_actual_1sat : Saturate  UpperLimit=255  LowerLimit=0
  Speeed_actual_Convert : DataTypeConversion  OutDataTypeStr=uint8
  Speeed_actual_Convert1 : DataTypeConversion  OutDataTypeStr=uint32
  Speeed_actual_D : Product  Inputs=*/
  Speeed_actual_F : Constant  OutDataTypeStr=single
  Speeed_actual_L : simulink/Logic and Bit Operations/Bitwise Operator  logicop=AND  UseBitMask=on  BitMask=255  BitMaskRealWorld=Stored Integer
  Speeed_actual_O : Constant  Value=0  OutDataTypeStr=single
  Speeed_actual_S : ArithShift
  Speeed_actual_sat : Saturate  UpperLimit=30  LowerLimit=0
  Speeed_actual_st : Sum  Inputs=+-
  output1 : Outport
  wires:
  Speeed_actual/1 -> Speeed_actual_sat/1
  Speeed_actual_sat/1 -> Speeed_actual_st/1
  Speeed_actual_O/1 -> Speeed_actual_st/2
  Speeed_actual_st/1 -> Speeed_actual_D/1
  Speeed_actual_F/1 -> Speeed_actual_D/2
  Speeed_actual_D/1 -> Speeed_actualRon/1
  Speeed_actualRon/1 -> Speeed_actual_S/1
  Speeed_actual_S/1 -> Speeed_actual_1sat/1
  Speeed_actual_1sat/1 -> Speeed_actual_Convert1/1
  Speeed_actual_Convert1/1 -> Speeed_actual_L/1
  Speeed_actual_L/1 -> Speeed_actual_Convert/1
  Speeed_actual_Convert/1 -> output1/1

== system FSAC2021/ROUTING/TO_ACAN/DV_driving_dynamics_1/Speeed_target ==
  Speeed_target : Inport
  Speeed_targetRon : Rounding  Operator=round
  Speeed_target_1sat : Saturate  UpperLimit=255  LowerLimit=0
  Speeed_target_Convert : DataTypeConversion  OutDataTypeStr=uint8
  Speeed_target_Convert1 : DataTypeConversion  OutDataTypeStr=uint32
  Speeed_target_D : Product  Inputs=*/
  Speeed_target_F : Constant  OutDataTypeStr=single
  Speeed_target_L : simulink/Logic and Bit Operations/Bitwise Operator  logicop=AND  UseBitMask=on  BitMask=255  BitMaskRealWorld=Stored Integer
  Speeed_target_O : Constant  Value=0  OutDataTypeStr=single
  Speeed_target_S : ArithShift
  Speeed_target_sat : Saturate  UpperLimit=30  LowerLimit=0
  Speeed_target_st : Sum  Inputs=+-
  output2 : Outport
  wires:
  Speeed_target/1 -> Speeed_target_sat/1
  Speeed_target_sat/1 -> Speeed_target_st/1
  Speeed_target_O/1 -> Speeed_target_st/2
  Speeed_target_st/1 -> Speeed_target_D/1
  Speeed_target_F/1 -> Speeed_target_D/2
  Speeed_target_D/1 -> Speeed_targetRon/1
  Speeed_targetRon/1 -> Speeed_target_S/1
  Speeed_target_S/1 -> Speeed_target_1sat/1
  Speeed_target_1sat/1 -> Speeed_target_Convert1/1
  Speeed_target_Convert1/1 -> Speeed_target_L/1
  Speeed_target_L/1 -> Speeed_target_Convert/1
  Speeed_target_Convert/1 -> output2/1

== system FSAC2021/ROUTING/TO_ACAN/DV_driving_dynamics_1/Streeing_angle_actual ==
  Streeing_angle_actual : Inport
  Streeing_angle_actualABS : Abs
  Streeing_angle_actualCS : ArithShift  BitShiftNumber=-8
  Streeing_angle_actualConS : Constant  OutDataTypeStr=single
  Streeing_angle_actualCosR : Constant  Value=0  OutDataTypeStr=uint8
  Streeing_angle_actualROP : RelationalOperator  Operator=<  OutDataTypeStr=boolean
  Streeing_angle_actualRon : Rounding  Operator=round
  Streeing_angle_actualSW : Switch  Criteria=u2 ~= 0
  Streeing_angle_actual_1sat : Saturate  UpperLimit=255  LowerLimit=0
  Streeing_angle_actual_Convert : DataTypeConversion  OutDataTypeStr=uint8
  Streeing_angle_actual_Convert1 : DataTypeConversion  OutDataTypeStr=uint32
  Streeing_angle_actual_D : Product  Inputs=*/
  Streeing_angle_actual_F : Constant  Value=0.5  OutDataTypeStr=single
  Streeing_angle_actual_L : simulink/Logic and Bit Operations/Bitwise Operator  logicop=AND  UseBitMask=on  BitMask=255  BitMaskRealWorld=Stored Integer
  Streeing_angle_actual_O : Constant  Value=-120  OutDataTypeStr=single
  Streeing_angle_actual_S : ArithShift
  Streeing_angle_actual_sat : Saturate  UpperLimit=120  LowerLimit=120
  Streeing_angle_actual_st : Sum  Inputs=+-
  Streeing_angle_actualsubcon : Sum  Inputs=+-
  output3 : Outport
  wires:
  Streeing_angle_actual/1 -> Streeing_angle_actual_sat/1
  Streeing_angle_actual_sat/1 -> Streeing_angle_actual_st/1
  Streeing_angle_actual_O/1 -> Streeing_angle_actual_st/2
  Streeing_angle_actual_st/1 -> Streeing_angle_actual_D/1
  Streeing_angle_actual_F/1 -> Streeing_angle_actual_D/2
  Streeing_angle_actual_D/1 -> Streeing_angle_actualRon/1
  Streeing_angle_actualRon/1 -> Streeing_angle_actualROP/1, Streeing_angle_actualABS/1, Streeing_angle_actualSW/3
  Streeing_angle_actualCosR/1 -> Streeing_angle_actualROP/2
  Streeing_angle_actualConS/1 -> Streeing_angle_actualCS/1
  Streeing_angle_actualCS/1 -> Streeing_angle_actualsubcon/1
  Streeing_angle_actualABS/1 -> Streeing_angle_actualsubcon/2
  Streeing_angle_actualsubcon/1 -> Streeing_angle_actualSW/1
  Streeing_angle_actualROP/1 -> Streeing_angle_actualSW/2
  Streeing_angle_actualSW/1 -> Streeing_angle_actual_S/1
  Streeing_angle_actual_S/1 -> Streeing_angle_actual_1sat/1
  Streeing_angle_actual_1sat/1 -> Streeing_angle_actual_Convert1/1
  Streeing_angle_actual_Convert1/1 -> Streeing_angle_actual_L/1
  Streeing_angle_actual_L/1 -> Streeing_angle_actual_Convert/1
  Streeing_angle_actual_Convert/1 -> output3/1

== system FSAC2021/ROUTING/TO_ACAN/DV_driving_dynamics_1/Streeing_angle_target ==
  Streeing_angle_target : Inport
  Streeing_angle_targetABS : Abs
  Streeing_angle_targetCS : ArithShift  BitShiftNumber=-8
  Streeing_angle_targetConS : Constant  OutDataTypeStr=single
  Streeing_angle_targetCosR : Constant  Value=0  OutDataTypeStr=uint8
  Streeing_angle_targetROP : RelationalOperator  Operator=<  OutDataTypeStr=boolean
  Streeing_angle_targetRon : Rounding  Operator=round
  Streeing_angle_targetSW : Switch  Criteria=u2 ~= 0
  Streeing_angle_target_1sat : Saturate  UpperLimit=255  LowerLimit=0
  Streeing_angle_target_Convert : DataTypeConversion  OutDataTypeStr=uint8
  Streeing_angle_target_Convert1 : DataTypeConversion  OutDataTypeStr=uint32
  Streeing_angle_target_D : Product  Inputs=*/
  Streeing_angle_target_F : Constant  Value=0.5  OutDataTypeStr=single
  Streeing_angle_target_L : simulink/Logic and Bit Operations/Bitwise Operator  logicop=AND  UseBitMask=on  BitMask=255  BitMaskRealWorld=Stored Integer
  Streeing_angle_target_O : Constant  Value=-120  OutDataTypeStr=single
  Streeing_angle_target_S : ArithShift
  Streeing_angle_target_sat : Saturate  UpperLimit=120  LowerLimit=-120
  Streeing_angle_target_st : Sum  Inputs=+-
  Streeing_angle_targetsubcon : Sum  Inputs=+-
  output4 : Outport
  wires:
  Streeing_angle_target/1 -> Streeing_angle_target_sat/1
  Streeing_angle_target_sat/1 -> Streeing_angle_target_st/1
  Streeing_angle_target_O/1 -> Streeing_angle_target_st/2
  Streeing_angle_target_st/1 -> Streeing_angle_target_D/1
  Streeing_angle_target_F/1 -> Streeing_angle_target_D/2
  Streeing_angle_target_D/1 -> Streeing_angle_targetRon/1
  Streeing_angle_targetRon/1 -> Streeing_angle_targetROP/1, Streeing_angle_targetABS/1, Streeing_angle_targetSW/3
  Streeing_angle_targetCosR/1 -> Streeing_angle_targetROP/2
  Streeing_angle_targetConS/1 -> Streeing_angle_targetCS/1
  Streeing_angle_targetCS/1 -> Streeing_angle_targetsubcon/1
  Streeing_angle_targetABS/1 -> Streeing_angle_targetsubcon/2
  Streeing_angle_targetsubcon/1 -> Streeing_angle_targetSW/1
  Streeing_angle_targetROP/1 -> Streeing_angle_targetSW/2
  Streeing_angle_targetSW/1 -> Streeing_angle_target_S/1
  Streeing_angle_target_S/1 -> Streeing_angle_target_1sat/1
  Streeing_angle_target_1sat/1 -> Streeing_angle_target_Convert1/1
  Streeing_angle_target_Convert1/1 -> Streeing_angle_target_L/1
  Streeing_angle_target_L/1 -> Streeing_angle_target_Convert/1
  Streeing_angle_target_Convert/1 -> output4/1

== system FSAC2021/ROUTING/TO_ACAN/DV_driving_dynamics_2/Acceleration_lateral ==
  Acceleration_lateral : Inport
  Acceleration_lateralABS : Abs
  Acceleration_lateralCOV : DataTypeConversion  OutDataTypeStr=uint8
  Acceleration_lateralCS : ArithShift  BitShiftNumber=-16
  Acceleration_lateralConS : Constant  OutDataTypeStr=single
  Acceleration_lateralCosR : Constant  Value=0  OutDataTypeStr=uint8
  Acceleration_lateralROP : RelationalOperator  Operator=<  OutDataTypeStr=boolean
  Acceleration_lateralRon : Rounding  Operator=round
  Acceleration_lateralSW : Switch  Criteria=u2 ~= 0
  Acceleration_lateral_1sat : Saturate  UpperLimit=65535  LowerLimit=0
  Acceleration_lateral_And : simulink/Logic and Bit Operations/Bitwise Operator  logicop=AND  UseBitMask=off  NumInputPorts=2  BitMask=bin2dec('11011001')  BitMaskRealWorld=Stored Integer
  Acceleration_lateral_And_C : Constant  Value=255  OutDataTypeStr=uint32
  Acceleration_lateral_Convert : DataTypeConversion  OutDataTypeStr=uint32
  Acceleration_lateral_D : Product  Inputs=*/
  Acceleration_lateral_D1 : Product  Inputs=*/
  Acceleration_lateral_F : Constant  Value=0.001953125  OutDataTypeStr=single
  Acceleration_lateral_L : simulink/Logic and Bit Operations/Bitwise Operator  logicop=AND  UseBitMask=on  BitMask=65535  BitMaskRealWorld=Stored Integer
  Acceleration_lateral_O : Constant  Value=0  OutDataTypeStr=single
  Acceleration_lateral_S : ArithShift
  Acceleration_lateral_sat : Saturate  UpperLimit=63.998046875  LowerLimit=-64
  Acceleration_lateral_st : Sum  Inputs=+-
  Acceleration_lateraloutput6_C : Constant  Value=256
  Acceleration_lateralsubcon : Sum  Inputs=+-
  BitCov : DataTypeConversion  OutDataTypeStr=uint8
  output5 : Outport
  output6 : Outport  Port=2
  wires:
  Acceleration_lateral/1 -> Acceleration_lateral_sat/1
  Acceleration_lateral_sat/1 -> Acceleration_lateral_st/1
  Acceleration_lateral_O/1 -> Acceleration_lateral_st/2
  Acceleration_lateral_st/1 -> Acceleration_lateral_D/1
  Acceleration_lateral_F/1 -> Acceleration_lateral_D/2
  Acceleration_lateral_D/1 -> Acceleration_lateralRon/1
  Acceleration_lateralRon/1 -> Acceleration_lateralROP/1, Acceleration_lateralABS/1, Acceleration_lateralSW/3
  Acceleration_lateralCosR/1 -> Acceleration_lateralROP/2
  Acceleration_lateralConS/1 -> Acceleration_lateralCS/1
  Acceleration_lateralCS/1 -> Acceleration_lateralsubcon/1
  Acceleration_lateralABS/1 -> Acceleration_lateralsubcon/2
  Acceleration_lateralsubcon/1 -> Acceleration_lateralSW/1
  Acceleration_lateralROP/1 -> Acceleration_lateralSW/2
  Acceleration_lateralSW/1 -> Acceleration_lateral_S/1
  Acceleration_lateral_S/1 -> Acceleration_lateral_1sat/1
  Acceleration_lateral_1sat/1 -> Acceleration_lateral_Convert/1
  Acceleration_lateral_Convert/1 -> Acceleration_lateral_L/1
  Acceleration_lateral_L/1 -> Acceleration_lateral_D1/1, Acceleration_lateral_And/1
  Acceleration_lateraloutput6_C/1 -> Acceleration_lateral_D1/2
  Acceleration_lateral_D1/1 -> Acceleration_lateralCOV/1
  Acceleration_lateralCOV/1 -> output6/1
  Acceleration_lateral_And_C/1 -> Acceleration_lateral_And/2
  Acceleration_lateral_And/1 -> BitCov/1
  BitCov/1 -> output5/1

== system FSAC2021/ROUTING/TO_ACAN/DV_driving_dynamics_2/Acceleration_longitudinal ==
  Acceleration_longitudinal : Inport
  Acceleration_longitudinalABS : Abs
  Acceleration_longitudinalCOV : DataTypeConversion  OutDataTypeStr=uint8
  Acceleration_longitudinalCS : ArithShift  BitShiftNumber=-16
  Acceleration_longitudinalConS : Constant  OutDataTypeStr=single
  Acceleration_longitudinalCosR : Constant  Value=0  OutDataTypeStr=uint8
  Acceleration_longitudinalROP : RelationalOperator  Operator=<  OutDataTypeStr=boolean
  Acceleration_longitudinalRon : Rounding  Operator=round
  Acceleration_longitudinalSW : Switch  Criteria=u2 ~= 0
  Acceleration_longitudinal_1sat : Saturate  UpperLimit=65535  LowerLimit=0
  Acceleration_longitudinal_And : simulink/Logic and Bit Operations/Bitwise Operator  logicop=AND  UseBitMask=off  NumInputPorts=2  BitMask=bin2dec('11011001')  BitMaskRealWorld=Stored Integer
  Acceleration_longitudinal_And_C : Constant  Value=255  OutDataTypeStr=uint32
  Acceleration_longitudinal_Convert : DataTypeConversion  OutDataTypeStr=uint32
  Acceleration_longitudinal_D : Product  Inputs=*/
  Acceleration_longitudinal_D1 : Product  Inputs=*/
  Acceleration_longitudinal_F : Constant  Value=0.001953125  OutDataTypeStr=single
  Acceleration_longitudinal_L : simulink/Logic and Bit Operations/Bitwise Operator  logicop=AND  UseBitMask=on  BitMask=65535  BitMaskRealWorld=Stored Integer
  Acceleration_longitudinal_O : Constant  Value=0  OutDataTypeStr=single
  Acceleration_longitudinal_S : ArithShift
  Acceleration_longitudinal_sat : Saturate  UpperLimit=63.998046875  LowerLimit=-64
  Acceleration_longitudinal_st : Sum  Inputs=+-
  Acceleration_longitudinaloutput2_C : Constant  Value=256
  Acceleration_longitudinalsubcon : Sum  Inputs=+-
  BitCov : DataTypeConversion  OutDataTypeStr=uint8
  output1 : Outport
  output2 : Outport  Port=2
  wires:
  Acceleration_longitudinal/1 -> Acceleration_longitudinal_sat/1
  Acceleration_longitudinal_sat/1 -> Acceleration_longitudinal_st/1
  Acceleration_longitudinal_O/1 -> Acceleration_longitudinal_st/2
  Acceleration_longitudinal_st/1 -> Acceleration_longitudinal_D/1
  Acceleration_longitudinal_F/1 -> Acceleration_longitudinal_D/2
  Acceleration_longitudinal_D/1 -> Acceleration_longitudinalRon/1
  Acceleration_longitudinalRon/1 -> Acceleration_longitudinalROP/1, Acceleration_longitudinalABS/1, Acceleration_longitudinalSW/3
  Acceleration_longitudinalCosR/1 -> Acceleration_longitudinalROP/2
  Acceleration_longitudinalConS/1 -> Acceleration_longitudinalCS/1
  Acceleration_longitudinalCS/1 -> Acceleration_longitudinalsubcon/1
  Acceleration_longitudinalABS/1 -> Acceleration_longitudinalsubcon/2
  Acceleration_longitudinalsubcon/1 -> Acceleration_longitudinalSW/1
  Acceleration_longitudinalROP/1 -> Acceleration_longitudinalSW/2
  Acceleration_longitudinalSW/1 -> Acceleration_longitudinal_S/1
  Acceleration_longitudinal_S/1 -> Acceleration_longitudinal_1sat/1
  Acceleration_longitudinal_1sat/1 -> Acceleration_longitudinal_Convert/1
  Acceleration_longitudinal_Convert/1 -> Acceleration_longitudinal_L/1
  Acceleration_longitudinal_L/1 -> Acceleration_longitudinal_D1/1, Acceleration_longitudinal_And/1
  Acceleration_longitudinaloutput2_C/1 -> Acceleration_longitudinal_D1/2
  Acceleration_longitudinal_D1/1 -> Acceleration_longitudinalCOV/1
  Acceleration_longitudinalCOV/1 -> output2/1
  Acceleration_longitudinal_And_C/1 -> Acceleration_longitudinal_And/2
  Acceleration_longitudinal_And/1 -> BitCov/1
  BitCov/1 -> output1/1
